simulink model "SS_HDS"  (R2019b)
settings: Solver=VariableStepAuto  StartTime=0.0  StopTime=60.0  FixedStep=0.00000001  RelTol=1e-3
undefined symbols (not defined in the file): __PRM__SERIALIZED__DATA__, HDS, SubsystemReferenceBlock
libraries: simulink x2, vrlib x1
settings Model: Creator=toons  LastModifiedBy=toons
settings DataIOCC: ExternalInput=[input1, input2]  ReturnWorkspaceOutputs=off
settings DebuggingCC: ArithmeticOperatorsInVariantConditions=warning
settings SFSimCC: CustomCodeUndefinedFunction=UseInterfaceOnly

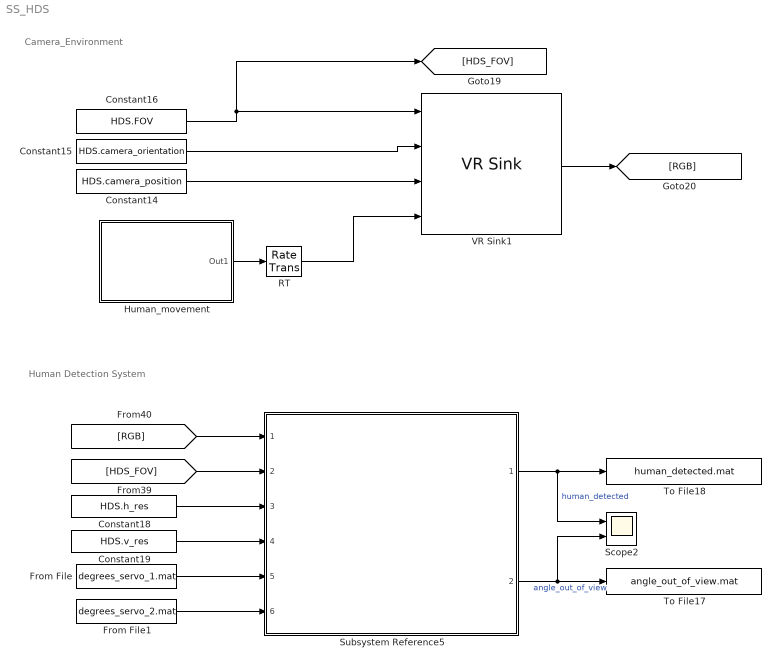
== system SS_HDS ==
  note: Camera_Environment
  note: Human Detection System
  Constant14 : Constant  Value=HDS.camera_position  VectorParams1D=off
  Constant15 : Constant  Value=HDS.camera_orientation  VectorParams1D=off
  Constant16 : Constant  Value=HDS.FOV  VectorParams1D=off
  Constant18 : Constant  Value=HDS.h_res  VectorParams1D=off
  Constant19 : Constant  Value=HDS.v_res  VectorParams1D=off
  From File : FromFile  FileName=degrees_servo_1.mat  SampleTime=1/30  ExtrapolationBeforeFirstDataPoint=Ground value  InterpolationWithinTimeRange=Zero order hold  ExtrapolationAfterLastDataPoint=Hold last value
  From File1 : FromFile  FileName=degrees_servo_2.mat  SampleTime=1/30  ExtrapolationBeforeFirstDataPoint=Hold first value  InterpolationWithinTimeRange=Zero order hold  ExtrapolationAfterLastDataPoint=Ground value
  "Human_movement " : Subsystem
  RT : RateTransition  OutPortSampleTime=0.1
  Scope2 : Scope  NumInputPorts=2
  Subsystem Reference5 : Subsystem  BlockKeywords=__PRM__SERIALIZED__DATA__:SubsystemReferenceBlock  ReferencedSubsystem=HDS_Detector
  To File17 : ToFile  Filename=angle_out_of_view.mat  SaveFormat=Timeseries
  To File18 : ToFile  Filename=human_detected.mat  SaveFormat=Timeseries
  VR Sink1 : vrlib/VR Sink  InstantiateOnLoad=on  SampleTime=0.1  ViewEnable=on  RemoteChange=off  RemoteView=off  FieldsWritten=Camera.fieldOfView.1.1.1.double#Camera.orientation.4.1.1.double#Camera.position.3.1.1.double#Human.translation.3.1.1.double  WorldFileName=HDS_Room_rotated.wrl  AutoView=off  VideoDimensions=[480 640]  AllowVariableSize=off
      settings: SourceProductBaseCode=VR
  wires:
  From File1/1 -> Subsystem Reference5/6
  Constant14/1 -> VR Sink1/3
  Constant15/1 -> VR Sink1/2
  Constant16/1 -> VR Sink1/1, [HDS_FOV]
  VR Sink1/1 -> [RGB]
  Constant19/1 -> Subsystem Reference5/4
  Constant18/1 -> Subsystem Reference5/3
  [RGB] -> Subsystem Reference5/1
  [HDS_FOV] -> Subsystem Reference5/2
  Subsystem Reference5/1 -> Scope2/1, To File18/1  "human_detected"
  Subsystem Reference5/2 -> To File17/1, Scope2/2  "angle_out_of_view"
  "Human_movement "/1(Out1) -> RT/1
  RT/1 -> VR Sink1/4
  From File/1 -> Subsystem Reference5/5

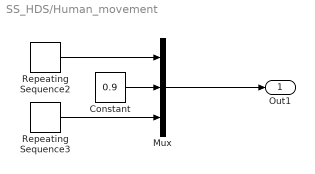
== system SS_HDS/Human_movement  ==
  Constant : Constant  Value=0.9
  Mux : Mux  Inputs=3
  Repeating Sequence2 : simulink/Sources/Repeating Sequence  rep_seq_t=[0 3 4 7 8 11 12 15 16]  rep_seq_y=[1 3.5 3.5 6 6 3.5 3.5 1 1]
  Repeating Sequence3 : simulink/Sources/Repeating Sequence  rep_seq_t=[0 3 4 7 8 11 12 15 16]  rep_seq_y=[0 -2.5 -2.5 0 0 2.5 2.5 0 0]
  Out1 : Outport  VectorParamsAs1DForOutWhenUnconnected=off
  wires:
  Mux/1 -> Out1/1
  Constant/1 -> Mux/2
  Repeating Sequence2/1 -> Mux/1
  Repeating Sequence3/1 -> Mux/3
